simulink model "PILTest1"  (Simulink 8.1)
settings: Solver=FixedStepDiscrete  StartTime=0.0  StopTime=10.0  RelTol=1e-3
undefined symbols (not defined in the file or in its folder): A14, B, B13, D, L3, R10
libraries: BAMLIB564xL x4, simulink_extras x3, rappid_564xl_ec_toolbox x2
settings Model: Creator=r61406  LastModifiedBy=evarshavskaya
settings DataIOCC: ExternalInput=off  InitialState=off  SaveOutput=off  SignalLogging=off  SaveTime=off
settings OptimizationCC: InlineParams=on  OptimizeModelRefInitCode=on  LifeSpan=1
settings DebuggingCC: InheritedTsInSrcMsg=none  SingleTaskRateTransMsg=error  ParameterDowncastMsg=none  ParameterOverflowMsg=warning  ParameterPrecisionLossMsg=none  ParameterTunabilityLossMsg=none  UnconnectedInputMsg=error  UnconnectedOutputMsg=error  UnconnectedLineMsg=error  UnknownTsInhSupMsg=error
settings HardwareCC: ProdLargestAtomicInteger=Long  ProdLargestAtomicFloat=Double  ProdIntDivRoundTo=Zero  ProdEndianess=BigEndian  ProdHWDeviceType=Freescale->32-bit PowerPC  TargetIntDivRoundTo=Zero  TargetEndianess=BigEndian  TargetHWDeviceType=Generic->Custom
settings RTWCC: SystemTargetFile=rappid564xl.tlc  MakeCommand=rappid_564xl_make_rtw  TemplateMakefile=rappid_564xl_default_tmf  PostCodeGenCommand=rappid_analyzegencode(buildInfo)  Description=RAppID Toolbox MPC564xL Code Generation Target (rappid)  ProcessScript=rappid564xl_make_rtw_hook  CreateSILPILBlock=PIL
settings CodeAppCC: IgnoreCustomStorageClasses=off  MaxIdLength=63  CustomSymbolStrType=$N$R$M  InternalIdentifier=Classic
settings STFCustomTargetCC: CodeReplacementLibrary=ANSI_C  CombineOutputUpdateFcns=on  SuppressErrorStatus=on  ERTCustomFileBanners=on  SupportAbsoluteTime=off  SupportContinuousTime=off  SupportNonInlinedSFcns=off  MATLABClassNameForMDSCustomization=Simulink.SoftwareTarget.ERTCustomization  GRTInterface=off  SystemTargetFile=rappid564xl.tlc
settings ERTTargetCC: CodeReplacementLibrary=ANSI_C  MultiwordLength=2048  ParMdlRefBuildCompliant=off  CompOptLevelCompliant=off  ConcurrentExecutionCompliant=off  SuppressErrorStatus=on  ERTFirstTimeCompliant=off  SupportAbsoluteTime=off  ModelStepFunctionPrototypeControlCompliant=off  CPPClassGenCompliant=off  InlinedParameterPlacement=NonHierarchical  ERTCustomFileTemplate=example_file_process.tlc  ConvertIfToSwitch=off  SuppressUnreachableDefaultCases=off

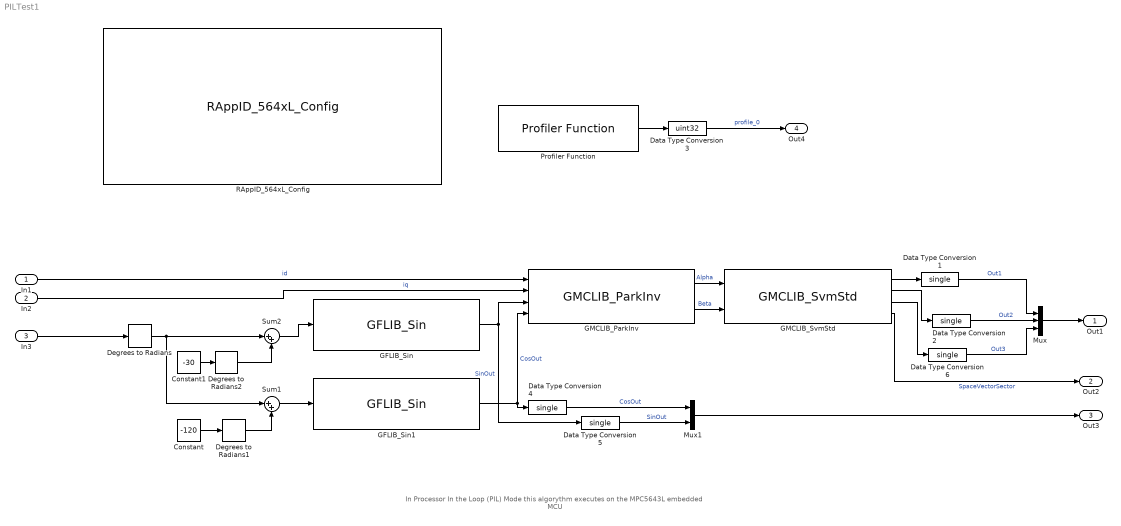
== system PILTest1 ==
  note: In Processor In the Loop (PIL) Mode this algorythm executes on the MPC5643L embedded MCU
  In1 : Inport
  In2 : Inport  Port=2
  In3 : Inport  Port=3
  Constant : Constant  Value=-120  OutDataTypeStr=single
  Constant1 : Constant  Value=-30  OutDataTypeStr=single
  Data Type Conversion{1..2,4..6} (5 alike) : DataTypeConversion  OutDataTypeStr=single
  Data Type Conversion3 : DataTypeConversion  OutDataTypeStr=uint32
  Degrees to Radians : simulink_extras/Transformations/Degrees to Radians
  Degrees to Radians1 : simulink_extras/Transformations/Degrees to Radians
  Degrees to Radians2 : simulink_extras/Transformations/Degrees to Radians
  GFLIB_Sin : BAMLIB564xL/General Functions/GFLIB_Sin
  GFLIB_Sin1 : BAMLIB564xL/General Functions/GFLIB_Sin
  GMCLIB_ParkInv : BAMLIB564xL/General Motor Control Functions/GMCLIB_ParkInv
  GMCLIB_SvmStd : BAMLIB564xL/General Motor Control Functions/GMCLIB_SvmStd
  Mux : Mux  Inputs=3
  Mux1 : Mux  Inputs=2
  "Profiler Function " : rappid_564xl_ec_toolbox/MPC564xL/Utility Blocks/Profiler Function   Priority=1  profile_indx=0
      settings: showOut=on
  RAppID_564xL_Config : rappid_564xl_ec_toolbox/MPC564xL/RAppID_564xL_Config  SystemClock=120  XTAL=40  MC_clock_60=12  MC_clock_80=16  MC_clock_120=10  SWG_clock_60=20  SWG_clock_80=13.334  SWG_clock_120=20  Compiler=GreenHills  MemTarget=RAM  Part=MPC5643L  Package=144 LQFP  global_int_priority=8  base_tick_priority=10  sys_task_supress=off  exception_handlers=off  stored_mdl_name=PILTest1  freemaster_interface=Oops  freemaster_rx_pin="LINFlex_0 Rx Pin 116 : \"PB[3]\""  freemaster_tx_pin="LINFlex_0 Tx Pin 114 : \"PB[2]\""  freemaster_interface_1=None  freemaster_enable=off  freemaster_rate=115200  freemaster_tx0_pin=18 : B[2] : 114 : A14  freemaster_rx0_pin=19 : B[3] : 116 : B13  freemaster_tx1_pin=57 : D[9] : 26 : L3  freemaster_rx1_pin=29 : B[13] : 60 : R10  freemaster_can_channel=1CH  freemater_can_speed=500K  freemaster_can_msgig=0x7AA  ccp_interface=None  ccp_enable=off  ccp_can_channel=CH1 (MB 0 - 1)  ccp_can_speed=500K  ccp_can_cro_id=256  ccp_can_dto_id=257  ccp_dev_id=RappID  ccp_dev_addr=0  ccp_odt=3  ccp_daq=3  pil_enable=on  pil_bam=off  comport=1  pil_rate=115200  bam_password_def=on  bam_password=0xFEEDFACECAFEBEEF  bam_sa_cs=off  bam_start_address=0x0  bam_code_size=0x7000  cons_dspi=on  cons_can=on  cons_adc=on  cons_pwm=on  cons_ctu=on  cons_swg=on  cons_eTimer=on  cons_fm=on
  Sum1 : Sum  Inputs=|++
  Sum2 : Sum  Inputs=|++
  Out1 : Outport
  Out2 : Outport  Port=2
  Out3 : Outport  Port=3
  Out4 : Outport  Port=4
  wires:
  GMCLIB_ParkInv/1 -> GMCLIB_SvmStd/1  "Alpha"
  GMCLIB_ParkInv/2 -> GMCLIB_SvmStd/2  "Beta"
  GMCLIB_SvmStd/1 -> Data Type Conversion1/1
  GMCLIB_SvmStd/2 -> Data Type Conversion2/1
  GMCLIB_SvmStd/3 -> Data Type Conversion6/1
  GMCLIB_SvmStd/4 -> Out2/1  "SpaceVectorSector"
  In1/1 -> GMCLIB_ParkInv/1  "id"
  GFLIB_Sin1/1 -> GMCLIB_ParkInv/4, Data Type Conversion4/1  "CosOut"
  GFLIB_Sin/1 -> GMCLIB_ParkInv/3, Data Type Conversion5/1  "SinOut"
  In2/1 -> GMCLIB_ParkInv/2  "iq"
  Mux/1 -> Out1/1
  Mux1/1 -> Out3/1
  Data Type Conversion1/1 -> Mux/1  "Out1"
  Data Type Conversion2/1 -> Mux/2  "Out2"
  Data Type Conversion6/1 -> Mux/3  "Out3"
  Data Type Conversion5/1 -> Mux1/2  "SinOut"
  Data Type Conversion4/1 -> Mux1/1  "CosOut"
  "Profiler Function "/1 -> Data Type Conversion3/1
  Data Type Conversion3/1 -> Out4/1  "profile_0"
  In3/1 -> Degrees to Radians/1
  Degrees to Radians/1 -> Sum2/1, Sum1/1
  Constant/1 -> Degrees to Radians1/1
  Degrees to Radians1/1 -> Sum1/2
  Constant1/1 -> Degrees to Radians2/1
  Degrees to Radians2/1 -> Sum2/2
  Sum2/1 -> GFLIB_Sin/1
  Sum1/1 -> GFLIB_Sin1/1
